simulink model "SlidingModeControl"  (R2021a)
settings: configuration reference "RPi_ControlRate" (kept outside this file)
settings Model: Creator=Andy  LastModifiedBy=Andy
settings ConfigSetRef: SourceName=RPi_ControlRate  SourceLocation=Base Workspace

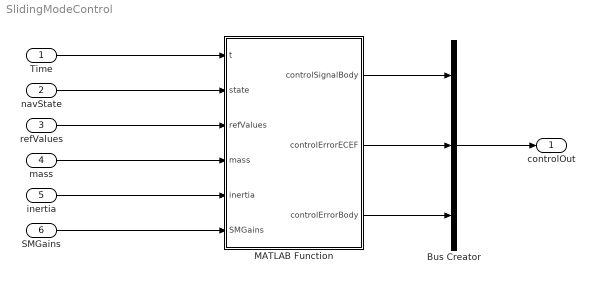
== system SlidingModeControl ==
  Time : Inport
  navState : Inport  Port=2  PortDimensions=12
  refValues : Inport  Port=3  PortDimensions=12
  mass : Inport  Port=4
  inertia : Inport  Port=5
  SMGains : Inport  Port=6  PortDimensions=9
  Bus Creator : BusCreator  Inputs=3  OutDataTypeStr=Bus: ControlOutBus
      settings: InheritFromInputs=off
  MATLAB Function : MATLAB Function  TreatAsAtomicUnit=on
  controlOut : Outport  OutDataTypeStr=Bus: ControlOutBus  VectorParamsAs1DForOutWhenUnconnected=off
  wires:
  Time/1 -> MATLAB Function/1(t)
  refValues/1 -> MATLAB Function/3(refValues)
  mass/1 -> MATLAB Function/4(mass)
  inertia/1 -> MATLAB Function/5(inertia)
  navState/1 -> MATLAB Function/2(state)
  MATLAB Function/2(controlErrorECEF) -> Bus Creator/2
  MATLAB Function/1(controlSignalBody) -> Bus Creator/1
  Bus Creator/1 -> controlOut/1
  MATLAB Function/3(controlErrorBody) -> Bus Creator/3
  SMGains/1 -> MATLAB Function/6(SMGains)

== matlab function SlidingModeControl/MATLAB Function ==
  data: t input; controlSignalBody output; state input; refValues input; mass input; inertia input; controlErrorECEF output; controlErrorBody output; SMGains input
function [controlSignalBody,controlErrorECEF,controlErrorBody] = callslidingModeControl(t,state,refValues,mass,inertia,SMGains)

 [controlSignalBody,controlErrorECEF,controlErrorBody] = slidingModeControl(t,state,refValues,mass,inertia,SMGains);
